simulink model "SMCFinalSim"  (R2024a)
settings: Solver=VariableStepAuto  StartTime=0.0  StopTime=15  RelTol=1e-3
undefined symbols (not defined in the file): a, beta, betaF, g, J, Kf, Lb, Lm, m_b, m_m
libraries: simulink_extras x1
settings Model: Creator=Cami  LastModifiedBy=alfar

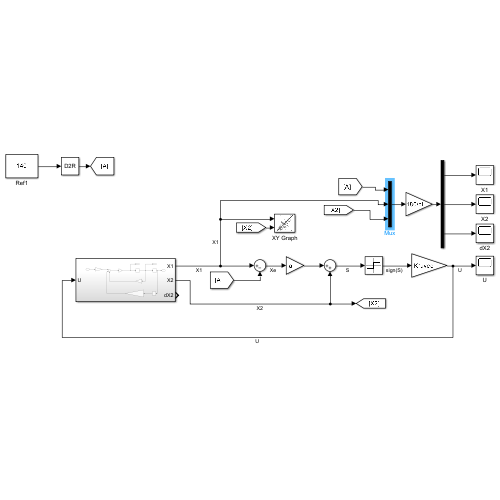
[thumbnail: Simulink's stored preview of the top-level diagram]
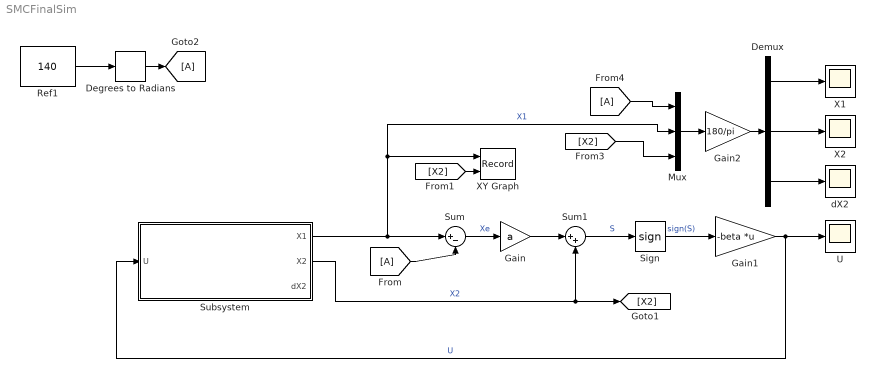
== system SMCFinalSim ==
  Degrees to Radians : simulink_extras/Transformations/Degrees to Radians
  Demux : Demux  Outputs=3
  From : From
  From4 : From
  Gain : Gain  Gain=a
  Gain1 : Gain  Gain=-beta  Multiplication=Matrix(K*u) (u vector)
  Gain2 : Gain  Gain=180/pi
  Goto2 : Goto
  Mux : Mux  Inputs=3
  Ref1 : Constant  Value=140
  Sign : Signum  ZeroCross=off
  Subsystem : Subsystem
  Sum : Sum  Inputs=|+-
  Sum1 : Sum  Inputs=|++
  U : Scope
  X1 : Scope
  X2 : Scope
  XY Graph : Record  FileSettingsInternal="{\"entries\":[{\"content\":{\"excelSettings\":{\"content\":{},\"type\":\"Streamout.ExcelSettings\"}},\"type\":\"Streamout.FileSettingStorage\",\"uuid\":\"\"}],\"packageUris\":[\"http:\\/\\/schema.mathworks.com\\/mf0\\/streamout_blocks\\/R2020a\"],\"version\":\"1.0\"}"  Layout=[1 1]  SignalsInternal="{\"entries\":[{\"content\":{\"signals\":[{\"content\":{\"blockPath\":[],\"dimensions\":[1],\"domain\":\"\",\"lineColor\":\"#a2142f\",\"plots\":[ 1 ],\"port\":1,\"sid\":[\"\"],\"signalID\":1,\"signalName\":\"X1\"},\"type\":\"RecordBlkView.Signal\",\"uuid\":\"\"},{\"content\":{\"blockPath\":[],\"dimensions\":[1],\"domain\":\"\",\"lineColor\":\"#139fff\",\"plots\":[ 1 ],\"port\":2,\"sid\":[\"\"],\"signalID\":2,\"signalName\":\"From1\"},\"type\":\"RecordBlkView.Signal\",\"uuid\":\"\"}]},\"type\":\"RecordBlkView.InputSignals\",\"uuid\":\"\"}],\"packageUris\":[\"http:\\/\\/schema.mathworks.com\\/mf0\\/streamout_blocks\\/R2020a\"],\"version\":\"1.0\"}"  VisualizationBindings="{\"xyplotplugin\":{\"info\":[{\"series\":[{\"bindingParametersList\":[{\"parameter\":\"X-Axis\",\"signalID\":1,\"signalName\":\"X1\"},{\"parameter\":\"Y-Axis\",\"signalID\":2,\"signalName\":\"From1\"}],\"seriesID\":0}],\"subplotID\":1}]}}"  CompatibilityTag=XY
  dX2 : Scope
  wires:
  Demux/1 -> X1/1
  Mux/1 -> Gain2/1
  Sum/1 -> Gain/1  "Xe"
  From4/1 -> Mux/1
  Gain1/1 -> Subsystem/1(U), U/1  "U"
  [X2] -> Mux/3
  Demux/2 -> X2/1
  Sign/1 -> Gain1/1  "sign(S)"
  Gain2/1 -> Demux/1
  Sum1/1 -> Sign/1  "S"
  Gain/1 -> Sum1/1
  [X2] -> XY Graph/2
  Subsystem/2(X2) -> [X2], Sum1/2  "X2"
  Demux/3 -> dX2/1
  Subsystem/1(X1) -> Sum/1, Mux/2, XY Graph/1  "X1"
  From/1 -> Sum/2
  Ref1/1 -> Degrees to Radians/1
  Degrees to Radians/1 -> Goto2/1

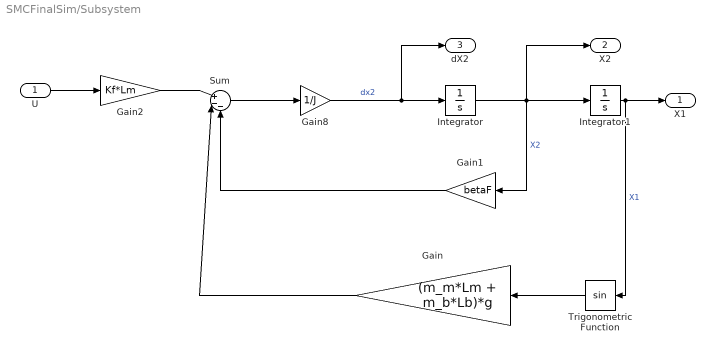
== system SMCFinalSim/Subsystem ==
  U : Inport
  Gain : Gain  Gain=(m_m*Lm + m_b*Lb)*g
  Gain1 : Gain  Gain=betaF
  Gain2 : Gain  Gain=Kf*Lm
  Gain8 : Gain  Gain=1/J
  Integrator : Integrator
  Integrator1 : Integrator
  Sum : Sum  Inputs=|+--
  Trigonometric Function : Trigonometry
  X1 : Outport
  X2 : Outport  Port=2
  dX2 : Outport  Port=3
  wires:
  U/1 -> Gain2/1
  Gain1/1 -> Sum/3
  Gain/1 -> Sum/2
  Gain2/1 -> Sum/1
  Integrator1/1 -> X1/1, Trigonometric Function/1  "X1"
  Trigonometric Function/1 -> Gain/1
  Sum/1 -> Gain8/1
  Integrator/1 -> X2/1, Gain1/1, Integrator1/1  "X2"
  Gain8/1 -> dX2/1, Integrator/1  "dx2"
